simulink model "sldemo_bangbang"  (Simulink 7.6)
settings: Solver=ode23  SolverMode=SingleTasking  StartTime=0.0  StopTime=100  MaxStep=0.1  RelTol=1e-6  AbsTol=1e-6
StartFcn:
  | if exist('hbbfig')
  |   if ishghandle(hbbfig,'figure')
  |     close(hbbfig)
  |   end
  |   clear hbbfig
  | end
StopFcn:
  | if ~exist('hbbfig')
  |   hbbfig = figure;
  | else
  |   set(0,'CurrentFigure', hbbfig);
  | end
  | if exist('x')
  |   plot(x(:,1),x(:,2)); grid
  |   shg;
  | end
Description:
  | State Events
  | 
  | This demonstrations shows state event handling.  Run the simulation and see the
  | phase plane plot, where the state x1 is along the X-axis and the state x2 is along
  | the Y-axis.
CloseFcn:
  | if exist('hbbfig')
  |   if ishghandle(hbbfig,'figure')
  |     close(hbbfig)
  |   end
  |   clear hbbfig
  |   if exist('x')
  |     clear x
  |   end
  |   if exist('t')
  |     clear t
  |   end
  | end
settings Model: Creator=The MathWorks Inc.  ExtModeAutoUpdateStatusClock=off
settings DataIOCC: ExternalInput=[]  InitialState=[]  LimitDataPoints=off  SaveOutput=off  SaveState=on  SignalLogging=off  StateSaveName=x  TimeSaveName=t
settings OptimizationCC: InlineInvariantSignals=on  InitFltsAndDblsToZero=on  BufferReusableBoundary=off
settings DebuggingCC: SaveWithParameterizedLinksMsg=none  SignalResolutionControl=TryResolveAllWithWarning  SolverPrmCheckMsg=none  MultiTaskDSMMsg=warning  MultiTaskCondExecSysMsg=none  BusObjectLabelMismatch=none
settings HardwareCC: TargetUnknown=on
settings RTWCC: IncludeERTFirstTime=on
settings CodeAppCC: CustomSymbolStrFcn=$F$N$M
settings GRTTargetCC: TargetFcnLib=ansi_tfl_tmw.mat

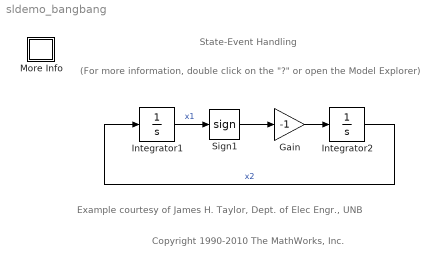
== system sldemo_bangbang ==
  note: State-Event Handling
  note: Example courtesy of James H. Taylor,
      | Dept. of Elec Engr., UNB
  note: (For more information, double click on
      | the "?" or open the Model Explorer)
  note: Copyright 1990-2010 The MathWorks, Inc.
  Gain : Gain  Gain=-1  SaturateOnIntegerOverflow=on  OutDataTypeStr=Inherit: Same as input  ParamDataTypeStr=Inherit: Same as input
  Integrator1 : Integrator  InitialCondition=0.25
  Integrator2 : Integrator  InitialCondition=0.25
  More Info : Subsystem
      settings: OpenFcn=showdemo(bdroot(gcs))
      mask Display: disp('?')
  Sign1 : Signum
  wires:
  Integrator2/1 -> Integrator1/1  "x2"
  Integrator1/1 -> Sign1/1  "x1"
  Sign1/1 -> Gain/1
  Gain/1 -> Integrator2/1

== system sldemo_bangbang/More Info ==
